simulink model "early_late_RC_48"  (R2014b)
settings: Solver=ode45  StartTime=0.0  StopTime=20000/fs  RelTol=1e-3
PreLoadFcn:
  | %%%%%%%%%%%%%%%%%%%%%%%%%%%%%%%%%%%%%%%%%%%%%%%%%%%%%%%%%%%%%%%%%%%%%%%%%%%
  | % check to see if Simulink library folder is missing from the MATLAB path %
  | %%%%%%%%%%%%%%%%%%%%%%%%%%%%%%%%%%%%%%%%%%%%%%%%%%%%%%%%%%%%%%%%%%%%%%%%%%%
  | if isempty(strfind(path, 'rtlsdr_book_library'))
  | 
  |     % create error window
  |     fig_error = figure(...
  |         'Name', 'Error: RTL-SDR Book Library',...
  |         'Toolbar','none',...
  |         'MenuBar','none',...
  |         'NumberTitle','off',...
  |         'Resize','off',...
  |         'WindowStyle','modal');
  |     fig_error.Position(3) = 600;
  |     fig_error.Position(4) = 150;
  |     fig_axes = axes(...
  |         'Parent',fig_error,...
  |         'Position',[0,0,1,1],...
  |         'visible','off');
  |     % error message
  |     t_title = text(.05,.8,...
  |         'MISSING DIRECTORIES',...
  |         'FontSize',11.5);
  |     t_body = text(.075,.6,...
  |         [{'Simulink cannot find the  \it{<root>}\rm / \it{rtlsdr\_book\_library}\rm  folder in the \it{MATLAB Path}\rm.'},...
  |         {'Please set the MATLAB path following the instructions given in Exercise 2.4.'}],...
  |         'FontSize',10.5);
  |     % buttons
  |     btn_path = uicontrol(...
  |         'Parent',fig_error,...
  |         'String','Set Path Now',...
  |         'FontSize',10,...
  |         'Callback', 'pathtool; close(fig_error);',...
  |         'Position', [fig_error.Position(3)/2-210, 30, 200, 30]);
  |     btn_abort = uicontrol(...
  |         'Parent',fig_error,...
  |         'String','No thanks',...
  |         'FontSize',10,...
  |         'Callback', 'close(fig_error); abort=1;',...
  |         'Position', [fig_error.Position(3)/2+10, 30, 200, 30]);
  | 
  |     % pause to allow user to interact with error box
  |     uiwait(fig_error);
  | 
  |     % abort simulation
  |     try
  |         if abort==1
  |             set_param(gcs, 'SimulationCommand', 'stop');
  |         end
  |     end
  | 
  |     % if user has set path, allow diagram to be updated
  |     if ~exist('abort','var')
  |         % create error window
  |         fig_update = figure(...
  |             'Name', 'Update Diagram',...
  |             'Toolbar','none',...
  |             'MenuBar','none',...
  |             'NumberTitle','off',...
  |             'Resize','off');
  |         fig_update.Position(3) = 400;
  |         fig_update.Position(4) = 120;
  |         fig_axes = axes(...
  |             'Parent',fig_update,...
  |             'Position',[0,0,1,1],...
  |             'visible','off');
  |         % instruction message
  |         t_body = text(.075,.7,...
  |             'Once you have set the path, update the block diagram',...
  |             'FontSize',10.5);
  |         % button
  |         btn_update = uicontrol(...
  |             'Parent',fig_update,...
  |             'String','Update Block Diagram',...
  |             'FontSize',10,...
  |             'Callback', 'set_param(gcs,''SimulationCommand'',''update''); close(gcf)',...
  |             'Position', [fig_update.Position(3)/2-100, 30, 200, 30]);
  |     end
  | 
  |     % clear error components
  |     clear('fig_error','fig_update','fig_axes','t_title','t_body','btn_path','btn_abort','btn_update','abort');
  | 
  | end
  | %%%%%%%%%%%%%%%%%%%%%%%%%%%%%%%%%%%%%%%%%%%%%%%%%%%%%%%%%%%%%%%%%%%%%%%%%%%
  | 
  | fs = 2.4e6;
  | 
  | Rdata = 100e3;
  | Rsymbol = Rdata/2;
  | interp = fs/Rsymbol;
  | %n_sym = samp/interp;
  | 
  | % ---------------- synch loop design ------------------
  | 
  | d = 0.707;                   % damping ratio
  | 
  | Ts = 1/Rsymbol;           % symbol period
  | Ks = 3.22;                    % phase detector coefficient
  | BnS = 0.1*Rsymbol;     % noise bandwidth in Hz
  | Kn   = 1;                     % gain of numerically controlled clock
  | 
  | % ------------ calculate loop filter coefficients -----------
  | 
  | Ka = (4*d*BnS*Ts)/(Kn*Ks*(d+1/(4*d)));
  | Kb = (4*(BnS*Ts)^2)/(Kn*Ks*(d+1/4*d)^2);
StopFcn:
  | figure(1)
  | hold off
  | plot(step_adj.time, step_adj.signals.values, 'b');
  | hold on
  | plot(step_nom.time, step_nom.signals.values, 'r');
  | xlabel('Time (s)');
  | ylabel('Amplitude');
  | legend('Adjusted Step Size','Quiescent Step Size','location','NorthEast');
  | setStandardFigSize(1);
  | set(1,'Name','Adjustment of Numerically Controlled Clock','NumberTitle','off');
  | 
  | 
  | % prepare for plotting
  | i_punctual_s = squeeze(i_punctual.signals.values);
  | q_punctual_s = squeeze(q_punctual.signals.values);
  | samples_s = squeeze(samples.signals.values);
  | 
  | sample_index = find(samples.signals.values ~= 0);
  | sig_samples = samples_s(sample_index);
  | sig_samples_t = samples.time(sample_index);
  | i_samp = i_punctual_s(sample_index);
  | q_samp = q_punctual_s(sample_index);
  | 
  | figure(2)
  | subplot(2,1,1)
  | hold off
  | plot(i_punctual.time, i_punctual_s,'g');
  | hold on
  | stem(sig_samples_t,(sig_samples.*i_samp),'b','MarkerFaceColor','b');
  | xlabel('Time');
  | ylabel('Amplitude');
  | legend('I punctual branch', 'Samples','location','NorthEast');
  | 
  | subplot(2,1,2)
  | hold off
  | plot(q_punctual.time, q_punctual_s,'m');
  | hold on
  | stem(sig_samples_t,(sig_samples.*q_samp),'b','MarkerFaceColor','b');
  | xlabel('Time');
  | ylabel('Amplitude');
  | legend('Q punctual branch', 'Samples','location','NorthEast');
  | 
  | setStandardFigSize(2);
  | set(2,'Name','Sampling of the I and Q Phases','NumberTitle','off');
undefined symbols (not defined in the file or in its folder): startfcn_constellation, startfcn_time_scope
libraries: simulink x5, commfilt2 x4, dsparch4 x2, rtlsdr_book_library x1, commrandsrc2 x1, commdigbbndpm3 x1
CloseFcn:
  | closefcn_model;
Description:
  | Software, Simulation Examples and Design Exercises Licence Agreement
  | 
  | This license agreement refers to the simulation examples, design exercises and files,
  | and associated software MATLAB and Simulink resources that accompany the book:
  | 
  |      Title: Software Defined Radio using MATLAB & Simulink and the RTL-SDR
  |      Published by Strathclyde Academic Media, 2015
  |      Authored by Robert W. Stewart, Kenneth W. Barlee, Dale S.W. Atkinson,
  |      and Louise H. Crockett
  | 
  | and made available as a download from, www.desktopSDR.com or variously acquired
  | by other means such as via USB storage, cloud storage, disk or any other electronic
  | or optical or magnetic storage mechanism. These files and associated software may
  | be used subject to the terms of agreement of the conditions below:
  | 
  |     Copyright © 2015 Robert W. Stewart, Kenneth W. Barlee, Dale S.W. Atkinson,
  |     and Louise H. Crockett
  |     All rights reserved.
  | 
  | Redistribution and use in source and binary forms, with or without modification, are
  | permitted provided that the following conditions are met:
  | 
  |    1.  Redistributions of source code must retain the above copyright notice, this list of
  |         conditions and the following disclaimer.
  | 
  |    2.  Redistributions in binary form must reproduce the above copyright notice, this
  |         list of conditions and the following disclaimer in the documentation and/or other
  |         materials provided with the distribution.
  | 
  |    3.  Neither the name of the copyright holder nor the names of its contributors may
  |         be used to endorse or promote products derived from this software without
  |         specific prior written permission.
  | 
  |    4.  In all cases, the software is, and all modifications and derivatives of the
  |         software shall be, licensed to you solely for use in conjunction with The
  |         MathWorks, Inc. products and service offerings.
  | 
  | THIS SOFTWARE IS PROVIDED BY THE COPYRIGHT HOLDERS AND CONTRIBUTORS
  | "AS IS" AND ANY EXPRESS OR IMPLIED WARRANTIES, INCLUDING, BUT NOT LIMITED
  | TO, THE IMPLIED WARRANTIES OF MERCHANTABILITY AND FITNESS FOR A
  | PARTICULAR PURPOSE ARE DISCLAIMED. IN NO EVENT SHALL THE COPYRIGHT
  | HOLDER OR CONTRIBUTORS BE LIABLE FOR ANY DIRECT, INDIRECT, INCIDENTAL,
  | SPECIAL, EXEMPLARY, OR CONSEQUENTIAL DAMAGES (INCLUDING, BUT NOT
  | LIMITED TO, PROCUREMENT OF SUBSTITUTE GOODS OR SERVICES; LOSS OF USE,
  | DATA, OR PROFITS; OR BUSINESS INTERRUPTION) HOWEVER CAUSED AND ON ANY
  | THEORY OF LIABILITY, WHETHER IN CONTRACT, STRICT LIABILITY, OR TORT
  | (INCLUDING NEGLIGENCE OR OTHERWISE) ARISING IN ANY WAY OUT OF THE USE
  | OF THIS SOFTWARE, EVEN IF ADVISED OF THE POSSIBILITY OF SUCH DAMAGE.
  | 
  | 
  | Audio Tracks used in Simulations Examples and Design Exercises
  | 
  | The music and vocal files used within the Examples files and software within the book
  | were variously written, arranged, performed, recorded and produced by Garrey Rice,
  | Adam Struth, Jamie Struth, Iain Thistlethwaite and also Marshall Craigmyle who
  | collectively, and individually where appropriate, assert and retain all of their copyright,
  | performance and artistic rights. Permission to use and reproduce this music is
  | granted for all purposes associated with MATLAB and Simulink software and the
  | simulation examples and design exercises files that accompany this book. Requests to
  | use the music for any other purpose should be directed to: info@desktopSDR.com.
  | For information on music track names, full credits, and links to the musicians please
  | refer to www.desktopSDR.com/more/audio.
settings Model: Creator=desktopSDR Team  LastModifiedBy=desktopSDR Team
settings DataIOCC: LimitDataPoints=off  SaveOutput=off  SignalLogging=off  SaveTime=off

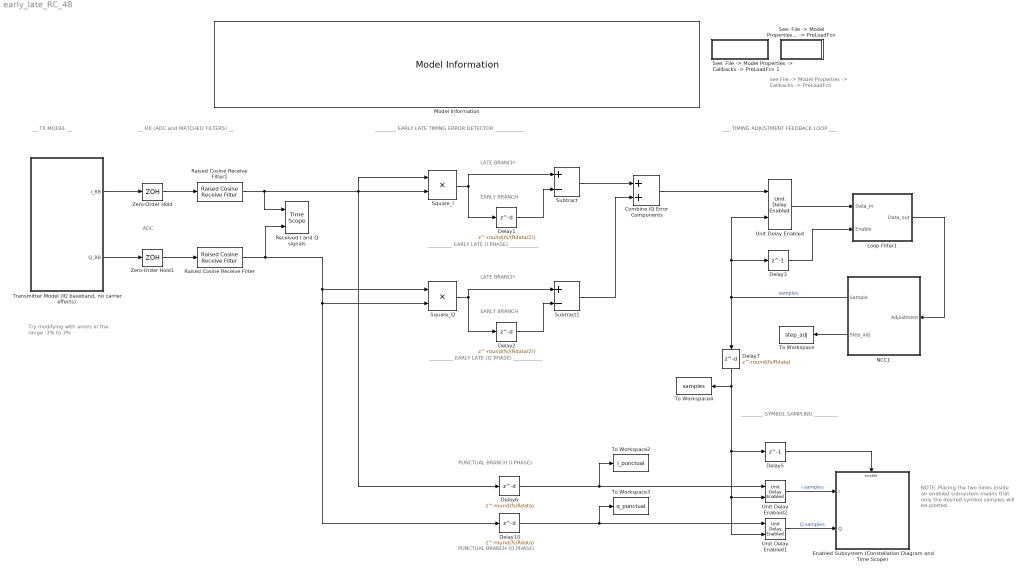
== system early_late_RC_48 ==
  note: Try modifying with errors
      | in the range -3% to 3%
  note: ADC
  note: NOTE:
      |
      | Placing the two Sinks inside an
      | enabled subsystem means that
      | only the desired symbol samples
      | will be plotted.
  note: ___ TIMING ADJUSTMENT FEEDBACK LOOP ___
  note: ________ EARLY LATE TIMING ERROR DETECTOR ___________
  note: LATE BRANCH
  note: EARLY BRANCH
  note: PUNCTUAL BRANCH (I PHASE)
  note: LATE BRANCH
  note: EARLY BRANCH
  note: _________ EARLY LATE (I PHASE) ___________
  note: _________ EARLY LATE (Q PHASE) ___________
  note: ________ SYMBOL SAMPLING _________
  note: PUNCTUAL BRANCH (Q PHASE)
  note: __ TX MODEL __
  note: __ RX (ADC and MATCHED FILTERS) __
  note: see File -> Model Properties
      | -> Callbacks -> PreLoadFcn
  Combine IQ Error Components : Sum
  Delay1 : Delay  DelayLength=round(fs/(Rdata/2))
  Delay10 : Delay  DelayLength=round(fs/Rdata)
  Delay2 : Delay  DelayLength=round(fs/(Rdata/2))
  Delay3 : Delay  DelayLength=1
  Delay5 : Delay  DelayLength=1
  Delay6 : Delay  DelayLength=round(fs/Rdata)
  Delay7 : Delay  DelayLength=round(fs/Rdata)
  Enabled Subsystem (Constellation Diagram and Time Scope) : Subsystem  TreatAsAtomicUnit=on
  Loop Filter1 : Subsystem
  Model Information : rtlsdr_book_library/Additional Tools/Model Information/Model Information
  NCC1 : Subsystem  mask(Numerically Controller Clock (NCC)){OSR=fs/Rsymbol}
      mask prompts: OSR "Oversampling Ratio"
      mask help:
      | This component operates similarly to a Numerically Controlled Oscillator (NCO).
      |
      | Internally, a nominal step size of (1 + Adjustment) is applied to an accumulator. The accumulator wraps around at N = OSR, therefore for a zero control input, the accumulator wraps once every symbol period at the expected rate.
      |
      | When the accumulator wraps, a strobe output is produced.
  Raised Cosine Receive Filter : commfilt2/Raised Cosine Receive Filter  filtType=Square root  N=interp  filtSpan=12  currentFiltSpan=12  D=(12)/2  R=0.5  sampMode=Mute  saveAsFlag=0  rateMode=Downsampling  downFactor=1  downOffset=0  framing=Allow multirate processing  checkGain=Normalized  filterGain=1  checkCoeff=off  variableName=rcRxFilt  launchFVT=on  roundingMode=Floor  overflowMode=off
  Raised Cosine Receive Filter1 : commfilt2/Raised Cosine Receive Filter  filtType=Square root  N=interp  filtSpan=12  currentFiltSpan=12  D=(12)/2  R=0.5  sampMode=Mute  saveAsFlag=0  rateMode=Downsampling  downFactor=1  downOffset=0  framing=Allow multirate processing  checkGain=Normalized  filterGain=1  checkCoeff=off  variableName=rcRxFilt1  launchFVT=on  roundingMode=Floor  overflowMode=off
  Received I and Q signals : TimeScope  StartFcn=startfcn_time_scope;  DefaultConfigurationName=spbscopes.TimeScopeBlockCfg  NumInputPorts=2
  "See: File -> Model Properties -> Callbacks -> PreLoadFcn " : Subsystem
      mask Display:
      | fs = evalin('base', 'fs');
      | fprintf(['fs = ',num2str(fs/1e6),' MHz']);
  "See: File -> Model Properties -> Callbacks -> PreLoadFcn 1" : Subsystem
      mask Display:
      | Rdata = evalin('base', 'Rdata');
      | fprintf(['Rdata = ',num2str(Rdata/1e3),' ksps']);
  Square_I : Product
  Square_Q : Product
  Subtract : Sum  Inputs=+-
  Subtract1 : Sum  Inputs=+-
  To Workspace : ToWorkspace  VariableName=step_adj  SaveFormat=Structure With Time  SampleTime=-1
  To Workspace2 : ToWorkspace  VariableName=i_punctual  SaveFormat=Structure With Time  SampleTime=-1
  To Workspace3 : ToWorkspace  VariableName=q_punctual  SaveFormat=Structure With Time  SampleTime=-1
  To Workspace4 : ToWorkspace  VariableName=samples  SaveFormat=Structure With Time  SampleTime=-1
  "Transmitter Model (IQ baseband, no carrier effects)" : Subsystem  mask(Transmitter Model (Baseband Data)){Error=-1}
      mask prompts: Error "% Timing Error"
      mask help: This transmitter block creates random QPSK data and applies RRC pulse shaping. The sample rate is adjusted based on the % timing error specified in the mask. The outputs from the block are analogue I and Q channels.
      mask init:
      | Offset = 1+(Error/100);
  Unit Delay Enabled : simulink/Additional Math & Discrete/Additional Discrete/Unit Delay Enabled  vinit=0.0  tsamp=-1
  Unit Delay Enabled1 : simulink/Additional Math & Discrete/Additional Discrete/Unit Delay Enabled  vinit=0.0  tsamp=-1
  Unit Delay Enabled2 : simulink/Additional Math & Discrete/Additional Discrete/Unit Delay Enabled  vinit=0.0  tsamp=-1
  Zero-Order Hold : ZeroOrderHold  SampleTime=1/(Rsymbol*interp)
  Zero-Order Hold1 : ZeroOrderHold  SampleTime=1/(Rsymbol*interp)
  wires:
  "Transmitter Model (IQ baseband, no carrier effects)"/2(Q_BB) -> Zero-Order Hold1/1
  "Transmitter Model (IQ baseband, no carrier effects)"/1(I_BB) -> Zero-Order Hold/1
  Zero-Order Hold/1 -> Raised Cosine Receive Filter1/1
  Zero-Order Hold1/1 -> Raised Cosine Receive Filter/1
  Square_I/1 -> Subtract/1, Delay1/1
  Delay1/1 -> Subtract/2
  Unit Delay Enabled/1 -> Loop Filter1/1(Data_in)
  NCC1/1(Sample) -> Unit Delay Enabled/2, Delay3/1, Delay7/1  "samples"
  Subtract/1 -> Combine IQ Error Components/1
  Delay3/1 -> Loop Filter1/2(Enable)
  Loop Filter1/1(Data_out) -> NCC1/1(Adjustment)
  Square_Q/1 -> Delay2/1, Subtract1/1
  Delay2/1 -> Subtract1/2
  Subtract1/1 -> Combine IQ Error Components/2
  Combine IQ Error Components/1 -> Unit Delay Enabled/1
  Raised Cosine Receive Filter1/1 -> Received I and Q signals/1, Square_I/1, Delay6/1, Square_I/2
  Raised Cosine Receive Filter/1 -> Delay10/1, Square_Q/2, Square_Q/1, Received I and Q signals/2
  Delay10/1 -> To Workspace3/1, Unit Delay Enabled1/1
  Delay6/1 -> To Workspace2/1, Unit Delay Enabled2/1
  Unit Delay Enabled2/1 -> Enabled Subsystem (Constellation Diagram and Time Scope)/1(I)  "I samples"
  Unit Delay Enabled1/1 -> Enabled Subsystem (Constellation Diagram and Time Scope)/2(Q)  "Q samples"
  Delay5/1 -> Enabled Subsystem (Constellation Diagram and Time Scope)/Enable
  NCC1/2(Step_adj) -> To Workspace/1
  Delay7/1 -> Delay5/1, Unit Delay Enabled2/2, Unit Delay Enabled1/2, To Workspace4/1

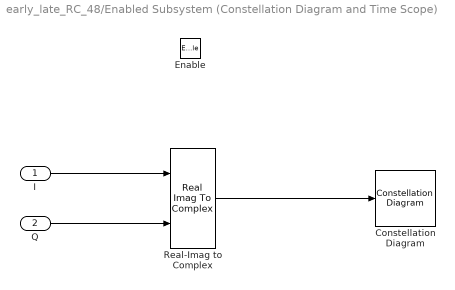
== system early_late_RC_48/Enabled Subsystem (Constellation Diagram and Time Scope) ==
  I : Inport
  Q : Inport  Port=2
  Enable : EnablePort
  Constellation Diagram : ConstellationDiagram  StartFcn=startfcn_constellation;
  Real-Imag to Complex : RealImagToComplex
  wires:
  I/1 -> Real-Imag to Complex/1
  Q/1 -> Real-Imag to Complex/2
  Real-Imag to Complex/1 -> Constellation Diagram/1

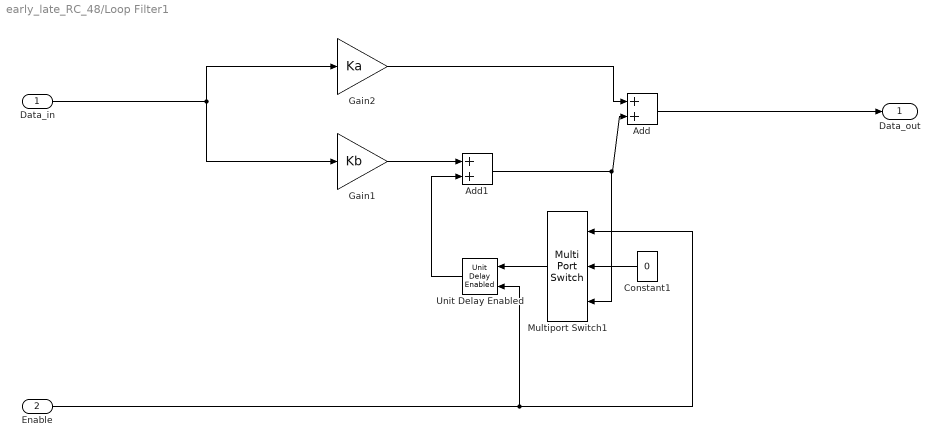
== system early_late_RC_48/Loop Filter1 ==
  Data_in : Inport
  Enable : Inport  Port=2
  Add : Sum
  Add1 : Sum
  Constant1 : Constant  Value=0  SampleTime=1/fs
  Gain1 : Gain  Gain=Kb
  Gain2 : Gain  Gain=Ka
  Multiport Switch1 : MultiPortSwitch  DataPortOrder=Zero-based contiguous  Inputs=2
  Unit Delay Enabled : simulink/Additional Math & Discrete/Additional Discrete/Unit Delay Enabled  vinit=0.0  tsamp=-1
  Data_out : Outport
  wires:
  Gain1/1 -> Add1/1
  Gain2/1 -> Add/1
  Unit Delay Enabled/1 -> Add1/2
  Add1/1 -> Multiport Switch1/3, Add/2
  Data_in/1 -> Gain2/1, Gain1/1
  Add/1 -> Data_out/1
  Enable/1 -> Unit Delay Enabled/2, Multiport Switch1/1
  Multiport Switch1/1 -> Unit Delay Enabled/1
  Constant1/1 -> Multiport Switch1/2

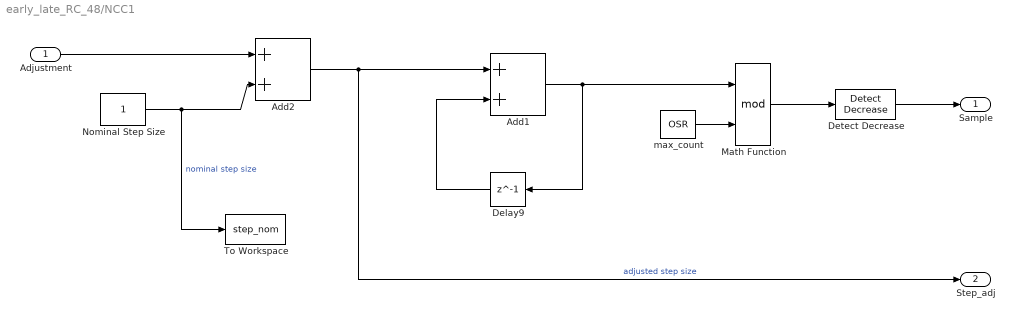
== system early_late_RC_48/NCC1 ==
  Adjustment : Inport
  Add1 : Sum  OutDataTypeStr=double
  Add2 : Sum  OutDataTypeStr=double
  Delay9 : Delay  DelayLength=1
  Detect Decrease : simulink/Logic and Bit Operations/Detect Decrease  vinit=0.0  InputProcessing=Inherited  OutDataTypeStr=boolean
  Math Function : Math  Operator=mod  SaturateOnIntegerOverflow=on
  Nominal Step Size : Constant  OutDataTypeStr=double  SampleTime=1/fs
  To Workspace : ToWorkspace  VariableName=step_nom  SaveFormat=Structure With Time  SampleTime=-1
  max_count : Constant  Value=OSR  OutDataTypeStr=double  SampleTime=1/fs
  Sample : Outport
  Step_adj : Outport  Port=2
  wires:
  Adjustment/1 -> Add2/1
  Add2/1 -> Step_adj/1, Add1/1  "adjusted step size"
  Delay9/1 -> Add1/2
  Nominal Step Size/1 -> To Workspace/1, Add2/2  "nominal step size"
  Add1/1 -> Delay9/1, Math Function/1
  Math Function/1 -> Detect Decrease/1
  max_count/1 -> Math Function/2
  Detect Decrease/1 -> Sample/1

== system early_late_RC_48/See: File -> Model Properties -> Callbacks -> PreLoadFcn  ==

== system early_late_RC_48/See: File -> Model Properties -> Callbacks -> PreLoadFcn 1 ==

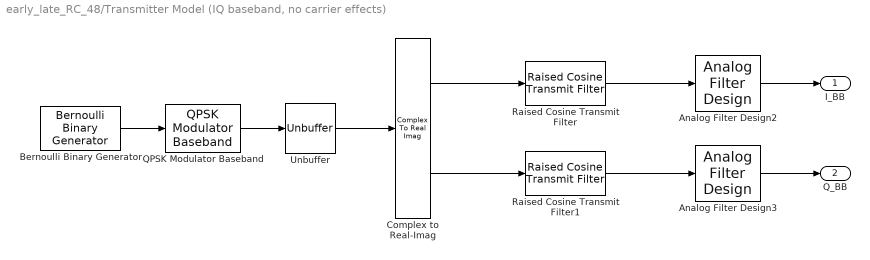
== system early_late_RC_48/Transmitter Model (IQ baseband, no carrier effects) ==
  Analog Filter Design2 : dsparch4/Analog Filter Design  method=Butterworth  filttype=Lowpass  N=8  Wlo=2*pi*Rsymbol*Offset  Whi=80  Rp=2  Rs=40
  Analog Filter Design3 : dsparch4/Analog Filter Design  method=Butterworth  filttype=Lowpass  N=8  Wlo=2*pi*Rsymbol*Offset  Whi=80  Rp=2  Rs=40
  Bernoulli Binary Generator : commrandsrc2/Bernoulli Binary Generator  P=0.5  seed=61  Ts=1/(Offset*Rdata)  frameBased=on  sampPerFrame=2  orient=off  outDataType=double
  Complex to Real-Imag : ComplexToRealImag
  QPSK Modulator Baseband : commdigbbndpm3/QPSK Modulator Baseband  InType=Bit  Enc=Gray  Ph=pi/4  outDtype=double  outWordLen=16  outUDDataType=sfix(16)  outFracLenMode=Best precision  outFracLen=15
  Raised Cosine Transmit Filter : commfilt2/Raised Cosine Transmit Filter  filtType=Square root  filtSpan=12  currentFiltSpan=12  D=(12)/2  R=0.5  sampMode=Mute  saveAsFlag=0  N=interp  framing=Allow multirate processing  checkGain=Normalized  filterGain=1  checkCoeff=off  variableName=rcTxFilt  launchFVT=on  roundingMode=Floor  overflowMode=off
  Raised Cosine Transmit Filter1 : commfilt2/Raised Cosine Transmit Filter  filtType=Square root  filtSpan=12  currentFiltSpan=12  D=(12)/2  R=0.5  sampMode=Mute  saveAsFlag=0  N=interp  framing=Allow multirate processing  checkGain=Normalized  filterGain=1  checkCoeff=off  variableName=rcTxFilt1  launchFVT=on  roundingMode=Floor  overflowMode=off
  Unbuffer : Unbuffer  SampleBasedProcessing=Same as frame based
  I_BB : Outport
  Q_BB : Outport  Port=2
  wires:
  Raised Cosine Transmit Filter1/1 -> Analog Filter Design3/1
  Unbuffer/1 -> Complex to Real-Imag/1
  Complex to Real-Imag/2 -> Raised Cosine Transmit Filter1/1
  Complex to Real-Imag/1 -> Raised Cosine Transmit Filter/1
  QPSK Modulator Baseband/1 -> Unbuffer/1
  Bernoulli Binary Generator/1 -> QPSK Modulator Baseband/1
  Analog Filter Design3/1 -> Q_BB/1
  Analog Filter Design2/1 -> I_BB/1
  Raised Cosine Transmit Filter/1 -> Analog Filter Design2/1
